simulink model "example_HeatExchanger"  (R2016b)
settings: Solver=ode23tb  StartTime=0.0  StopTime=1500  RelTol=1e-3  AbsTol=1e-6
libraries: carnot x5, simulink x1
Description:
  | % This file is part of the CARNOT Blockset.
  | %
  | % Copyright (c) 1998-2015, Solar-Institute Juelich of the FH Aachen.
  | % Additional Copyright for this file see list auf authors.
  | % All rights reserved.
  | %
  | % Redistribution and use in source and binary forms, with or without
  | % modification, are permitted provided that the following conditions are
  | % met:
  | %
  | % 1. Redistributions of source code must retain the above copyright notice,
  | %    this list of conditions and the following disclaimer.
  | %
  | % 2. Redistributions in binary form must reproduce the above copyright
  | %    notice, this list of conditions and the following disclaimer in the
  | %    documentation and/or other materials provided with the distribution.
  | %
  | % 3. Neither the name of the copyright holder nor the names of its
  | %    contributors may be used to endorse or promote products derived from
  | %    this software without specific prior written permission.
  | %
  | % THIS SOFTWARE IS PROVIDED BY THE COPYRIGHT HOLDERS AND CONTRIBUTORS "AS IS"
  | % AND ANY EXPRESS OR IMPLIED WARRANTIES, INCLUDING, BUT NOT LIMITED TO, THE
  | % IMPLIED WARRANTIES OF MERCHANTABILITY AND FITNESS FOR A PARTICULAR PURPOSE
  | % ARE DISCLAIMED. IN NO EVENT SHALL THE COPYRIGHT HOLDER OR CONTRIBUTORS BE
  | % LIABLE FOR ANY DIRECT, INDIRECT, INCIDENTAL, SPECIAL, EXEMPLARY, OR
  | % CONSEQUENTIAL DAMAGES (INCLUDING, BUT NOT LIMITED TO, PROCUREMENT OF
  | % SUBSTITUTE GOODS OR SERVICES; LOSS OF USE, DATA, OR PROFITS; OR BUSINESS
  | % INTERRUPTION) HOWEVER CAUSED AND ON ANY THEORY OF LIABILITY, WHETHER IN
  | % CONTRACT, STRICT LIABILITY, OR TORT (INCLUDING NEGLIGENCE OR OTHERWISE)
  | % ARISING IN ANY WAY OUT OF THE USE OF THIS SOFTWARE, EVEN IF ADVISED OF
  | % THE POSSIBILITY OF SUCH DAMAGE.
settings Model: ExtModeTrigMode=oneshot  ExtModeArmWhenConnect=off  Creator=drhf  LastModifiedBy=drhf
settings DataIOCC: SaveFormat=Array  SignalLoggingName=sigsOut
settings OptimizationCC: BooleanDataType=off  ExpressionDepthLimit=2147483647  InitFltsAndDblsToZero=on  LifeSpan=inf
settings DebuggingCC: SaveWithParameterizedLinksMsg=none  SignalResolutionControl=TryResolveAllWithWarning  MultiTaskDSMMsg=warning  MultiTaskCondExecSysMsg=none  StateNameClashWarn=warning  SFUnexpectedBacktrackingDiag=warning  SFNoUnconditionalDefaultTransitionDiag=warning  SFExecutionAtInitializationDiag=none
settings HardwareCC: ProdBitPerPointer=32  ProdBitPerSizeT=32  ProdBitPerPtrDiffT=32  ProdLargestAtomicFloat=None  ProdIntDivRoundTo=Undefined  ProdEndianess=Unspecified  ProdWordSize=32  ProdHWDeviceType=32-bit Generic  TargetUnknown=on
settings ModelReferenceCC: PropagateSignalLabelsOutOfModel=off
settings RTWCC: TemplateMakefile=grt_vc.tmf
settings GRTTargetCC: TargetFcnLib=ansi_tfl_tmw.mat  TargetLangStandard=C89/C90 (ANSI)  ModelReferenceCompliant=off  GeneratePreprocessorConditionals=Disable all  CombineOutputUpdateFcns=off  MatFileLogging=off  GRTInterface=on
settings ConfigComp: CovMetricSettings=dw  CovHtmlReporting=on  CovSaveCumulativeToWorkspaceVar=on  CovSaveSingleToWorkspaceVar=on  CovExternalEMLEnable=off

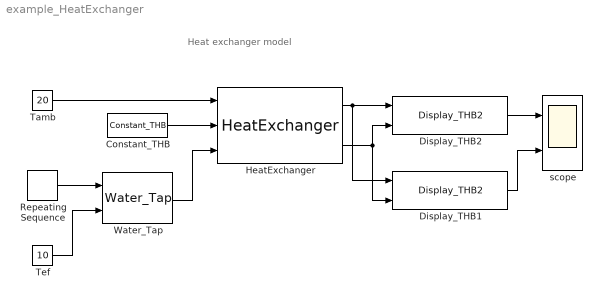
== system example_HeatExchanger ==
  note: Heat exchanger model
  Constant_THB : carnot/Source/Simple/Constant_THB  t=60  mdot=0.15  p=1e5  mID=No Pressure Drop  fluid=Water  mix=0  mix2=0  mix3=0  dia=0.02  hgt=0
  Display_THB1 : carnot/Outputs/Display_THB2  t=off  m=on  p=off  id=off  mix=off  d=off
  Display_THB2 : carnot/Outputs/Display_THB2  t=on  m=off  p=off  id=off  mix=off  d=off
  HeatExchanger : carnot/Source/Heat_Exchanger/HeatExchanger  flowtype=1  ua0=2000  uahot=[0.04 0]  uacold=[0.04 0]  ualoss=3  cap=10e3  linh=20  quah=10  linc=20  quac=10  t0=20
  Repeating Sequence : simulink/Sources/Repeating Sequence  rep_seq_t=[ 0 600 600+eps(600) 1200]  rep_seq_y=[ 0 0 0.2+0*eps(600) 0.2]
  Tamb : Constant  Value=20
  Tef : Constant  Value=10
  Water_Tap : carnot/Load/Hot_Water_Tapping/Water_Tap  dia=0.02  p=2e5
  scope : Scope  NumInputPorts=2
  wires:
  Constant_THB/1 -> HeatExchanger/2
  Tamb/1 -> HeatExchanger/1
  Water_Tap/1 -> HeatExchanger/3
  Repeating Sequence/1 -> Water_Tap/1
  Display_THB2/1 -> scope/1
  HeatExchanger/1 -> Display_THB2/1, Display_THB1/1
  HeatExchanger/2 -> Display_THB2/2, Display_THB1/2
  Tef/1 -> Water_Tap/2
  Display_THB1/1 -> scope/2
